simulink model "p2_p3"  (R2017a)
settings: Solver=VariableStepAuto  StartTime=0.0  StopTime=10.0  RelTol=1e-3
libraries: fl_lib x22, nesl_utility x10
settings Model: Creator=Jesus  LastModifiedBy=Jesus

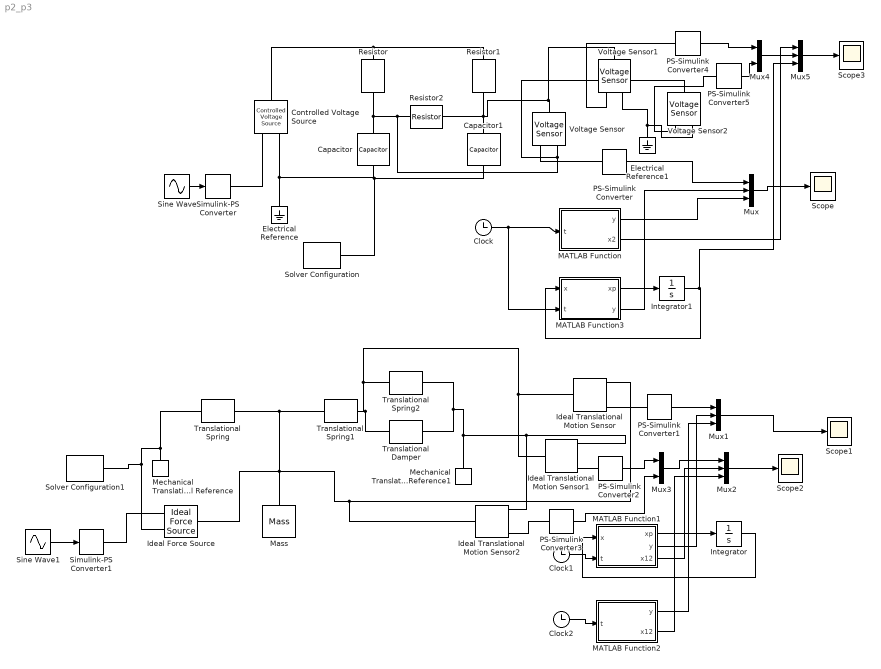
== system p2_p3 ==
  Capacitor : fl_lib/Electrical/Electrical Elements/Capacitor  c=1 F  r=1e-6 Ohm  g=0 1/Ohm  i_specify=off  i_priority=None  i=0 A  i_nominal_specify=off  i_nominal_unit=A  i_nominal_value=1  v_specify=off  v_priority=None  v=0 V  v_nominal_specify=off  v_nominal_unit=V  v_nominal_value=1  vc_specify=off  vc_priority=High  vc=0 V  vc_nominal_specify=off  vc_nominal_unit=V  vc_nominal_value=1
  Capacitor1 : fl_lib/Electrical/Electrical Elements/Capacitor  c=2 F  r=1e-6 Ohm  g=0 1/Ohm  i_specify=off  i_priority=None  i=0 A  i_nominal_specify=off  i_nominal_unit=A  i_nominal_value=1  v_specify=off  v_priority=None  v=0 V  v_nominal_specify=off  v_nominal_unit=V  v_nominal_value=1  vc_specify=off  vc_priority=High  vc=0 V  vc_nominal_specify=off  vc_nominal_unit=V  vc_nominal_value=1
  Clock : Clock
  Clock1 : Clock
  Clock2 : Clock
  Controlled Voltage Source : fl_lib/Electrical/Electrical Sources/Controlled Voltage Source
  Electrical Reference : fl_lib/Electrical/Electrical Elements/Electrical Reference
  Electrical Reference1 : fl_lib/Electrical/Electrical Elements/Electrical Reference
  Ideal Force Source : fl_lib/Mechanical/Mechanical Sources/Ideal Force Source
  Ideal Translational Motion Sensor : fl_lib/Mechanical/Mechanical Sensors/Ideal Translational Motion Sensor  offset=0 m
  Ideal Translational Motion Sensor1 : fl_lib/Mechanical/Mechanical Sensors/Ideal Translational Motion Sensor  offset=0 m
  Ideal Translational Motion Sensor2 : fl_lib/Mechanical/Mechanical Sensors/Ideal Translational Motion Sensor  offset=0 m
  Integrator : Integrator  InitialCondition=[0 0 0]
  Integrator1 : Integrator  InitialCondition=[0 0]
  MATLAB Function : MATLAB Function  TreatAsAtomicUnit=on
  MATLAB Function1 : MATLAB Function  TreatAsAtomicUnit=on
  MATLAB Function2 : MATLAB Function  TreatAsAtomicUnit=on
  MATLAB Function3 : MATLAB Function  TreatAsAtomicUnit=on
  Mass : fl_lib/Mechanical/Translational Elements/Mass  mass=10 kg  v_specify=off  v_priority=High  v=0 m/s  v_nominal_specify=off  v_nominal_unit=m/s  v_nominal_value=1  f_specify=off  f_priority=None  f=0 N  f_nominal_specify=off  f_nominal_unit=N  f_nominal_value=1
  Mechanical Translational Reference : fl_lib/Mechanical/Translational Elements/Mechanical Translational Reference
  Mechanical Translational Reference1 : fl_lib/Mechanical/Translational Elements/Mechanical Translational Reference
  Mux{,1..2,5} (4 alike) : Mux  Inputs=3
  Mux3 : Mux  Inputs=2
  Mux4 : Mux  Inputs=2
  PS-Simulink Converter{,1..5} (6 alike) : nesl_utility/PS-Simulink Converter  PhysicalDomain=network_engine_domain  SubClassName=ps_output  LeftPortType=input  RightPortType=output  PseudoPeriodic=off  Frequencies=[]  Unit=1  AffineConversion=off
  Resistor : fl_lib/Electrical/Electrical Elements/Resistor  R=5 Ohm  i_specify=off  i_priority=None  i=0 A  i_nominal_specify=off  i_nominal_unit=A  i_nominal_value=1  v_specify=off  v_priority=None  v=0 V  v_nominal_specify=off  v_nominal_unit=V  v_nominal_value=1
  Resistor1 : fl_lib/Electrical/Electrical Elements/Resistor  R=10 Ohm  i_specify=off  i_priority=None  i=0 A  i_nominal_specify=off  i_nominal_unit=A  i_nominal_value=1  v_specify=off  v_priority=None  v=0 V  v_nominal_specify=off  v_nominal_unit=V  v_nominal_value=1
  Resistor2 : fl_lib/Electrical/Electrical Elements/Resistor  R=1 Ohm  i_specify=off  i_priority=None  i=0 A  i_nominal_specify=off  i_nominal_unit=A  i_nominal_value=1  v_specify=off  v_priority=None  v=0 V  v_nominal_specify=off  v_nominal_unit=V  v_nominal_value=1
  Scope{,1..3} (4 alike) : Scope
  Simulink-PS Converter : nesl_utility/Simulink-PS Converter  PhysicalDomain=network_engine_domain  SubClassName=ps_input  LeftPortType=input  RightPortType=output  PseudoPeriodic=off  Frequencies=[]  NoiseDistribution=none  NoiseParameters=[]  Unit=1  AffineConversion=off  FilteringAndDerivatives=provide  SimscapeFilterOrder=1  InputFilterTimeConstant=0.001  UdotUserProvided=0
  Simulink-PS Converter1 : nesl_utility/Simulink-PS Converter  PhysicalDomain=network_engine_domain  SubClassName=ps_input  LeftPortType=input  RightPortType=output  PseudoPeriodic=off  Frequencies=[]  NoiseDistribution=none  NoiseParameters=[]  Unit=1  AffineConversion=off  FilteringAndDerivatives=provide  SimscapeFilterOrder=1  InputFilterTimeConstant=0.001  UdotUserProvided=0
  Sine Wave : Sin  Amplitude=10  SampleTime=0
  Sine Wave1 : Sin  SampleTime=0
  Solver Configuration : nesl_utility/Solver Configuration  PhysicalDomain=network_engine_domain  SubClassName=solver  LeftPortType=input  RightPortType=generic  Accelerate=off  Tones=[]  Harmonics=[]  SimulateNoise=off  Profile=off  UseLocalSampling=off  EnableSwitchedLinearOptims=on  FrequencyDomain=off  UseCCode=off  RelTol=0.001  AbsTol=1e-06  MinStep=1e-09  ToWorkspace=off  RevertToSquareIcSolve=off  NumHomotopyIterations=100  PhasorMode=off  PhasorModeNumHarmonics=1  OverrideAbsTol=off  DoDC=off  ResidualTolerance=1e-09  UseLocalSolver=off  LocalSolverChoice=NE_BACKWARD_EULER_ADVANCER  LocalSolverSampleTime=0.001  DoFixedCost=off  MaxNonlinIter=3  MaxModeIter=2  LinearAlgebra=Sparse  DelaysMemoryBudget=1024  AutomaticFiltering=on  FilteringTimeConstant=0.001
  Solver Configuration1 : nesl_utility/Solver Configuration  PhysicalDomain=network_engine_domain  SubClassName=solver  LeftPortType=input  RightPortType=generic  Accelerate=off  Tones=[]  Harmonics=[]  SimulateNoise=off  Profile=off  UseLocalSampling=off  EnableSwitchedLinearOptims=on  FrequencyDomain=off  UseCCode=off  RelTol=0.001  AbsTol=1e-06  MinStep=1e-09  ToWorkspace=off  RevertToSquareIcSolve=off  NumHomotopyIterations=100  PhasorMode=off  PhasorModeNumHarmonics=1  OverrideAbsTol=off  DoDC=off  ResidualTolerance=1e-09  UseLocalSolver=off  LocalSolverChoice=NE_BACKWARD_EULER_ADVANCER  LocalSolverSampleTime=0.001  DoFixedCost=off  MaxNonlinIter=3  MaxModeIter=2  LinearAlgebra=Sparse  DelaysMemoryBudget=1024  AutomaticFiltering=on  FilteringTimeConstant=0.001
  Translational Damper : fl_lib/Mechanical/Translational Elements/Translational Damper  D=.5 N/(m/s)  v_specify=off  v_priority=None  v=0 m/s  v_nominal_specify=off  v_nominal_unit=m/s  v_nominal_value=1  f_specify=off  f_priority=None  f=0 N  f_nominal_specify=off  f_nominal_unit=N  f_nominal_value=1
  Translational Spring : fl_lib/Mechanical/Translational Elements/Translational Spring  spr_rate=2 N/m  v_specify=off  v_priority=None  v=0 m/s  v_nominal_specify=off  v_nominal_unit=m/s  v_nominal_value=1  f_specify=off  f_priority=None  f=0 N  f_nominal_specify=off  f_nominal_unit=N  f_nominal_value=1  x_specify=off  x_priority=High  x=0 m  x_nominal_specify=off  x_nominal_unit=m  x_nominal_value=1
  Translational Spring1 : fl_lib/Mechanical/Translational Elements/Translational Spring  spr_rate=1 N/m  v_specify=off  v_priority=None  v=0 m/s  v_nominal_specify=off  v_nominal_unit=m/s  v_nominal_value=1  f_specify=off  f_priority=None  f=0 N  f_nominal_specify=off  f_nominal_unit=N  f_nominal_value=1  x_specify=off  x_priority=High  x=0 m  x_nominal_specify=off  x_nominal_unit=m  x_nominal_value=1
  Translational Spring2 : fl_lib/Mechanical/Translational Elements/Translational Spring  spr_rate=.5 N/m  v_specify=off  v_priority=None  v=0 m/s  v_nominal_specify=off  v_nominal_unit=m/s  v_nominal_value=1  f_specify=off  f_priority=None  f=0 N  f_nominal_specify=off  f_nominal_unit=N  f_nominal_value=1  x_specify=off  x_priority=High  x=0 m  x_nominal_specify=off  x_nominal_unit=m  x_nominal_value=1
  Voltage Sensor : fl_lib/Electrical/Electrical Sensors/Voltage Sensor
  Voltage Sensor1 : fl_lib/Electrical/Electrical Sensors/Voltage Sensor
  Voltage Sensor2 : fl_lib/Electrical/Electrical Sensors/Voltage Sensor
  wires:
  PS-Simulink Converter/1 -> Mux/1
  Sine Wave/1 -> Simulink-PS Converter/1
  Sine Wave1/1 -> Simulink-PS Converter1/1
  PS-Simulink Converter1/1 -> Mux1/1
  Mux1/1 -> Scope1/1
  MATLAB Function1/1(xp) -> Integrator/1
  Integrator/1 -> MATLAB Function1/1(x)
  Clock1/1 -> MATLAB Function1/2(t)
  MATLAB Function1/2(y) -> Mux1/2
  Clock2/1 -> MATLAB Function2/1(t)
  MATLAB Function2/1(y) -> Mux1/3
  Clock/1 -> MATLAB Function3/2(t), MATLAB Function/1(t)
  MATLAB Function3/1(xp) -> Integrator1/1
  Integrator1/1 -> Mux5/3, MATLAB Function3/1(x)
  Mux3/1 -> Mux2/1
  PS-Simulink Converter2/1 -> Mux3/1
  PS-Simulink Converter3/1 -> Mux3/2
  Mux2/1 -> Scope2/1
  MATLAB Function1/3(x12) -> Mux2/2
  MATLAB Function2/2(x12) -> Mux2/3
  PS-Simulink Converter4/1 -> Mux4/1
  PS-Simulink Converter5/1 -> Mux4/2
  Mux4/1 -> Mux5/1
  Mux5/1 -> Scope3/1
  MATLAB Function/2(x2) -> Mux5/2
  Mux/1 -> Scope/1
  MATLAB Function3/2(y) -> Mux/2
  MATLAB Function/1(y) -> Mux/3
  connections:
  Resistor1/LConn1 -- Controlled Voltage Source/LConn1 -- Resistor/LConn1
  Resistor2/LConn1 -- Voltage Sensor1/LConn1 -- Voltage Sensor/LConn1 -- Resistor1/RConn1 -- Capacitor1/LConn1
  Resistor2/RConn1 -- Voltage Sensor2/LConn1 -- Voltage Sensor/RConn2 -- Capacitor/LConn1 -- Resistor/RConn1
  Capacitor1/RConn1 -- Electrical Reference/LConn1 -- Controlled Voltage Source/RConn2 -- Solver Configuration/RConn1 -- Capacitor/RConn1
  Simulink-PS Converter/RConn1 -- Controlled Voltage Source/RConn1
  PS-Simulink Converter/LConn1 -- Voltage Sensor/RConn1
  Mass/LConn1 -- Ideal Translational Motion Sensor2/LConn1 -- Ideal Translational Motion Sensor/RConn1 -- Ideal Force Source/LConn1 -- Translational Spring1/LConn1 -- Translational Spring/RConn1
  Mechanical Translational Reference/LConn1 -- Solver Configuration1/RConn1 -- Ideal Force Source/RConn2 -- Translational Spring/LConn1
  Translational Spring2/LConn1 -- Ideal Translational Motion Sensor1/LConn1 -- Ideal Translational Motion Sensor/LConn1 -- Translational Damper/LConn1 -- Translational Spring1/RConn1
  Translational Spring2/RConn1 -- Ideal Translational Motion Sensor2/RConn1 -- Ideal Translational Motion Sensor1/RConn1 -- Mechanical Translational Reference1/LConn1 -- Translational Damper/RConn1
  Simulink-PS Converter1/RConn1 -- Ideal Force Source/RConn1
  PS-Simulink Converter1/LConn1 -- Ideal Translational Motion Sensor/RConn3
  PS-Simulink Converter2/LConn1 -- Ideal Translational Motion Sensor1/RConn3
  Ideal Translational Motion Sensor2/RConn3 -- PS-Simulink Converter3/LConn1
  Electrical Reference1/LConn1 -- Voltage Sensor2/RConn2 -- Voltage Sensor1/RConn2
  PS-Simulink Converter4/LConn1 -- Voltage Sensor1/RConn1
  PS-Simulink Converter5/LConn1 -- Voltage Sensor2/RConn1

== matlab function p2_p3/MATLAB Function1 ==
  data: xp output; x input; y output; t input; x12 output
function [xp,y,x12] = fcn(x,t)
k1=2;
k2=1;
k3=.5;
b1=.5;
m1=10;
u=sin(t);
A=[0,1,0;-(k1/m1)-(k2/m1),0,k2/m1;k2/b1,0,(-k2/b1)-(k3/b1)];
B=[0,1/m1,0]';
C=[-1,0,1];
xp=A*x+B*u;
x12=[x(1),x(3)]
y=C*x;

== matlab function p2_p3/MATLAB Function ==
  data: t input; y output; x2 output
function [y,x2] = fcn(t)
u=10*sin(t);
x1 =(440*sin(t))/769 - (6400*cos(t))/5383 + (6400*exp(-(7*t)/8)*(cosh((969^(1/2)*t)/40) + (21*969^(1/2)*sinh((969^(1/2)*t)/40))/1292))/5383; 
x2 =(4600*exp(-(7*t)/8)*(cosh((969^(1/2)*t)/40) + (313*969^(1/2)*sinh((969^(1/2)*t)/40))/7429))/5383 - (670*sin(t))/5383 - (4600*cos(t))/5383;

y=x2-x1;
x12=[x1, x2];

== matlab function p2_p3/MATLAB Function2 ==
  data: t input; y output; x12 output
function [y,x12] = fcn(t)

%y=75 - (1875*exp(-t/5))/26 - (75*cos(t))/26 - (245*sin(t))/26 - 5*t;
y=0.0022172472720731870193351994823803*exp(-2.9781888183120855013344827821287*t) + 0.027681660899653979238754325259516*cos(t) + 0.051903114186851211072664359861592*sin(t) - 0.029898908171727166258089524741896*exp(-0.010905590843957249332758608935638*t)*cos(0.48468881838889569804507542020527*t) - 0.094134208758088965502827713468213*exp(-0.010905590843957249332758608935638*t)*sin(0.48468881838889569804507542020527*t);
x1=0.000024447000534299612289796785289094*exp(-2.9781888183120855013344827821287*t) - 0.0034602076124567474048442906574394*cos(t) - 0.1314878892733564013840830449827*sin(t) + 0.0034357606119224477925544938721504*exp(-0.010905590843957249332758608935638*t)*cos(0.48468881838889569804507542020527*t) + 0.27151062921957282867439002308629*exp(-0.010905590843957249332758608935638*t)*sin(0.48468881838889569804507542020527*t);
x2=0.0022416942726074866316249962676694*exp(-2.9781888183120855013344827821287*t) + 0.024221453287197231833910034602076*cos(t) - 0.079584775086505190311418685121107*sin(t) - 0.026463147559804718465535030869746*exp(-0.010905590843957249332758608935638*t)*cos(0.48468881838889569804507542020527*t) + 0.17737642046148386317156230961807*exp(-0.010905590843957249332758608935638*t)*sin(0.48468881838889569804507542020527*t);
x12=[x1,x2];

== matlab function p2_p3/MATLAB Function3 ==
  data: xp output; x input; y output; t input
function [xp,y] = fcn(x,t)
u=10*sin(t);
A=[-6/5 1;1/2 -11/20];
B=[1/5 1/20]';
C=[-1 1];
xp=A*x+B*u;
y=C*x;
%y=y1(1)-.5*y1(2);
